simulink model "roboticSending"  (R2025b)
settings: Solver=FixedStepAuto  StartTime=0.0  StopTime=inf  RelTol=1e-3
model workspace (MAT data in the model file):
  SL_ROS_VariableLengthArrays_MaxSizes.CommonInfo.ArrayTruncateAction = 'EmitWarning'
  SL_ROS_VariableLengthArrays_MaxSizes.MsgTypeMap = containers.Map
  SL_ROS_VariableLengthArrays_MaxSizes.MsgTypeMap.serialization.keys = {'control_msgs/JointJog', 'sensor_msgs/JointState'}
  SL_ROS_VariableLengthArrays_MaxSizes.MsgTypeMap.serialization.values{1}(1).PropertyName = 'displacements'
  SL_ROS_VariableLengthArrays_MaxSizes.MsgTypeMap.serialization.values{1}(1).DataType = 'double'
  SL_ROS_VariableLengthArrays_MaxSizes.MsgTypeMap.serialization.values{1}(1).MaxLength = 6
  SL_ROS_VariableLengthArrays_MaxSizes.MsgTypeMap.serialization.values{1}(2).PropertyName = 'joint_names'
  SL_ROS_VariableLengthArrays_MaxSizes.MsgTypeMap.serialization.values{1}(2).DataType = 'std_msgs/String'
  SL_ROS_VariableLengthArrays_MaxSizes.MsgTypeMap.serialization.values{1}(2).MaxLength = 6
  SL_ROS_VariableLengthArrays_MaxSizes.MsgTypeMap.serialization.values{1}(3).PropertyName = 'velocities'
  SL_ROS_VariableLengthArrays_MaxSizes.MsgTypeMap.serialization.values{1}(3).DataType = 'double'
  SL_ROS_VariableLengthArrays_MaxSizes.MsgTypeMap.serialization.values{1}(3).MaxLength = 6
  SL_ROS_VariableLengthArrays_MaxSizes.MsgTypeMap.serialization.values{2}(1).PropertyName = 'effort'
  SL_ROS_VariableLengthArrays_MaxSizes.MsgTypeMap.serialization.values{2}(1).DataType = 'double'
  SL_ROS_VariableLengthArrays_MaxSizes.MsgTypeMap.serialization.values{2}(1).MaxLength = 6
  SL_ROS_VariableLengthArrays_MaxSizes.MsgTypeMap.serialization.values{2}(2).PropertyName = 'name'
  SL_ROS_VariableLengthArrays_MaxSizes.MsgTypeMap.serialization.values{2}(2).DataType = 'std_msgs/String'
  SL_ROS_VariableLengthArrays_MaxSizes.MsgTypeMap.serialization.values{2}(2).MaxLength = 6
  SL_ROS_VariableLengthArrays_MaxSizes.MsgTypeMap.serialization.values{2}(3).PropertyName = 'position'
  SL_ROS_VariableLengthArrays_MaxSizes.MsgTypeMap.serialization.values{2}(3).DataType = 'double'
  SL_ROS_VariableLengthArrays_MaxSizes.MsgTypeMap.serialization.values{2}(3).MaxLength = 6
  SL_ROS_VariableLengthArrays_MaxSizes.MsgTypeMap.serialization.values{2}(4).PropertyName = 'velocity'
  SL_ROS_VariableLengthArrays_MaxSizes.MsgTypeMap.serialization.values{2}(4).DataType = 'double'
  SL_ROS_VariableLengthArrays_MaxSizes.MsgTypeMap.serialization.values{2}(4).MaxLength = 6
  SL_ROS_VariableLengthArrays_MaxSizes.MsgTypeMap.serialization.uniformity = 0
  SL_ROS_VariableLengthArrays_MaxSizes.MsgTypeMap.serialization.keyType = 'char'
  SL_ROS_VariableLengthArrays_MaxSizes.MsgTypeMap.serialization.valueType = 'any'
values from neighbouring files (symbols this model uses):
  Error_threshold = 0.03    [RoboticCourseworkdata.sldd]
  Kd = 0.01    [RoboticCourseworkdata.sldd]
  Ki = 0.02    [RoboticCourseworkdata.sldd]
  Kp = 5.0    [RoboticCourseworkdata.sldd]
  Sample_time = 0.02    [RoboticCourseworkdata.sldd]
undefined symbols (not defined in the file or in its folder): DiscIntNeverNeededParam, Levenberg, Marquardt, velocities, velocities_SL_Info
libraries: ros2lib x3, robotmaniplib x2, robotcorelib x1, simulink_extras x1, simulink x1, SignalEditorBlockLib x1
settings Model: DataDictionary=RoboticCourseworkdata.sldd  Creator=jack  LastModifiedBy=jack
settings OptimizationCC: DefaultParameterBehavior=Inlined  EnhancedBackFolding=on  PassReuseOutputArgsAs=Individual arguments  ZeroExternalMemoryAtStartup=off  ZeroInternalMemoryAtStartup=off  MaxStackSize=64  OptimizeBlockOrder=speed  DifferentSizesBufferReuse=on  OptimizationCustomize=off  EfficientTunableParamExpr=on
settings DebuggingCC: ParameterTunabilityLossMsg=error
settings HardwareCC: ProdBitPerLong=64.0  ProdHWDeviceType=Intel->x86-64 (Linux 64)
settings SFSimCC: MATLABDynamicMemAlloc=off
settings RTWCC: SystemTargetFile=ert.tlc  HardwareBoard=Robot Operating System 2 (ROS 2)  TLCOptions="-aInlineSetEventsForThisBaseRateFcn=TLC_FALSE -aSuppressMultiTaskScheduler=TLC_FALSE  -aRateBasedStepFcn=0"  GenCodeOnly=on  TemplateMakefile=ert_default_tmf  Toolchain=Colcon Tools  TargetLang=C++  Description=Embedded Coder
settings CodeAppCC: ForceParamTrailComments=on  IgnoreCustomStorageClasses=off  OperatorAnnotations=on  SimulinkDataObjDesc=on  SFDataObjDesc=on  InsertBlockDesc=on
settings ERTTargetCC: ExtModeTransport=2.0  ExtModeStaticAlloc=on  ExtModeMexFile=ext_xcp  ExtModeIntrfLevel=Level2 - Open  RootIOFormat=Structure reference  CodeInterfacePackaging=C++ class

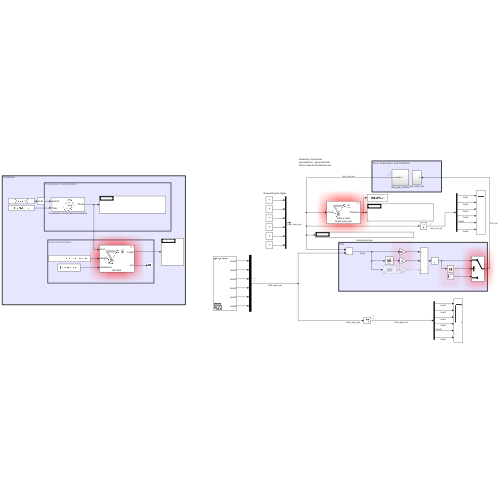
[thumbnail: Simulink's stored preview of the top-level diagram]
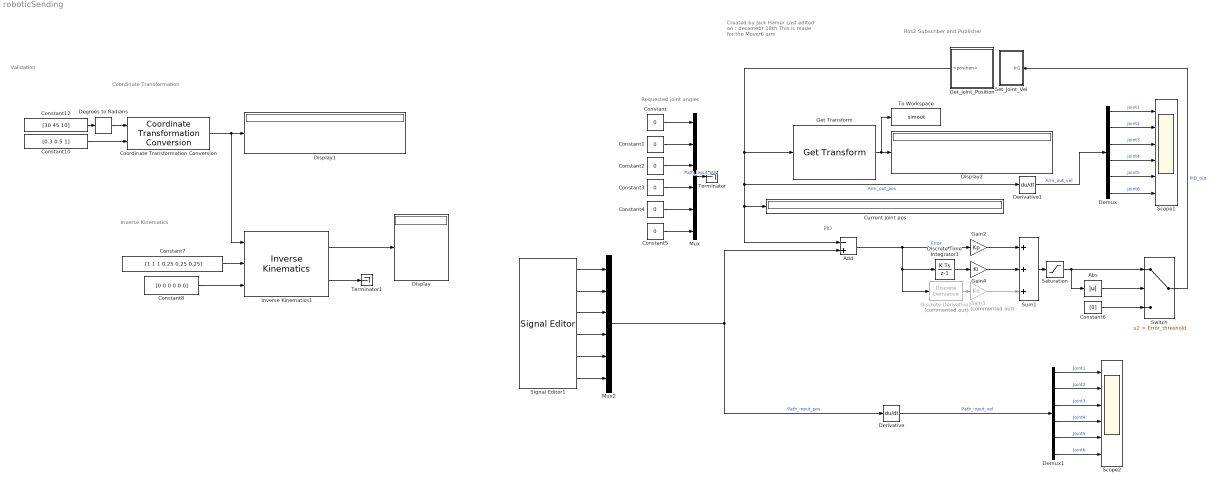
== system roboticSending ==
  note: Validation
  note: Created by Jack Hamer
      | Last edited on : decemebr 18th
      | This is made for the Mover6 arm
  note: Coordinate Transformation
  note: Inverse Kinematics
  note: PID
  note: Ros2 Subscriber and Publisher
  note: Requested joint angles
  Abs : Abs  SaturateOnIntegerOverflow=off
  Add : Sum  Inputs=-+
  Constant{,1..5} (6 alike) : Constant  Value=0
  Constant10 : Constant  Value=[0.3 0.5 1]
  Constant12 : Constant  Value=[30 45 10]
  Constant6 : Constant  Value=[0]  SampleTime=Sample_time
  Constant7 : Constant  Value=[1 1 1 0.25 0.25 0.25]
  Constant8 : Constant  Value=[0 0 0 0 0 0]
  Coordinate Transformation Conversion : robotcorelib/Coordinate Transformation Conversion  InputRepresentation=Euler Angles  InputEulerSequence=ZYX  ShowTrVecInputPort=on  OutputRepresentation=Homogeneous Transformation  OutputEulerSequence=ZYX  ShowTrVecOutputPort=on  SimulateUsing=Interpreted execution
  Current joint pos : Display
  Degrees to Radians : simulink_extras/Transformations/Degrees to Radians
  Demux : Demux  Outputs=6
  Demux1 : Demux  Outputs=6
  Derivative : Derivative
  Derivative1 : Derivative
  Discrete Derivative1 : simulink/Discrete/Discrete Derivative  Commented=on  gainval=1.0  ICPrevScaledInput=0.0  OutMin=[]  OutMax=[]  OutDataType=fixdt(1, 16)  OutScaling=2^-10  DoSatur=off
  Discrete-Time Integrator1 : DiscreteIntegrator  SampleTime=-1  ICPrevOutput=DiscIntNeverNeededParam  ICPrevScaledInput=DiscIntNeverNeededParam
  Display : Display
  Display1 : Display
  Display2 : Display
  Gain2 : Gain  Gain=Kp
  Gain3 : Gain  Commented=on  Gain=Kd
  Gain4 : Gain  Gain=Ki
  Get Transform : robotmaniplib/Get Transform  RigidBodyTree=Mover6import  SourceBody=link6  TargetBody=base_link  SimulateUsing=Interpreted execution
  Get_joint_Position : Subsystem
  Inverse Kinematics1 : robotmaniplib/Inverse Kinematics  RigidBodyTree=Mover6import  EndEffector=link6  ShowInfo=on  SolverName=Levenberg-Marquardt  EnforceJointLimits=on  MaxIterations=1500  MaxTime=10  GradientTolerance=1e-3  SolutionTolerance=1e-2  StepTolerance=1e-7  ConstraintTolerance=1e-6  ErrorChangeTolerance=1e-3  UseErrorDamping=on  DampingBias=0.0025  SimulateUsing=Interpreted execution
  Mux : Mux  Inputs=6
  Mux2 : Mux  Inputs=6
  Saturation : Saturate  UpperLimit=2  LowerLimit=-2
  Scope1 : Scope  NumInputPorts=6
      settings: ActiveDisplayYMinimum=-3.329826235975621  ActiveDisplayYMaximum=3.372443564924636
  Scope2 : Scope  NumInputPorts=6
      settings: ActiveDisplayYMinimum=-1.9531250848653292  ActiveDisplayYMaximum=2.2527181340884104
  Set_Joint_Vel : Subsystem
  Signal Editor1 : SignalEditorBlockLib/Signal Editor  FileName=TrapzodialControlsig.mat  ActiveScenario=path_senario  ActiveSignal=Joint1  IsBus=off  OutputBusObjectStr=Bus: BusObject  SampleTime=0  ZeroCross=off  OutputAfterFinalValue=Holding final value  Unit=inherit  PreserveSignalName=on  ApplySigPropsToAllScenarios=on  ApplySigPropsToAllSignals=on  SignalPropertySource=Dialog parameters
  Sum1 : Sum  Inputs=+++
  Switch : Switch  Criteria=u2 > Threshold  Threshold=Error_threshold  SaturateOnIntegerOverflow=off  InputSameDT=off
  Terminator : Terminator
  Terminator1 : Terminator
  To Workspace : ToWorkspace  VariableName=simout  SaveFormat=Timeseries  SampleTime=-1
  wires:
  Saturation/1 -> Switch/1, Abs/1
  Sum1/1 -> Saturation/1
  Gain2/1 -> Sum1/1
  Add/1 -> Discrete Derivative1/1, Discrete-Time Integrator1/1, Gain2/1  "Error"
  Discrete-Time Integrator1/1 -> Gain4/1
  Gain4/1 -> Sum1/2
  Gain3/1 -> Sum1/3
  Discrete Derivative1/1 -> Gain3/1
  Constant/1 -> Mux/1
  Constant1/1 -> Mux/2
  Constant2/1 -> Mux/3
  Constant5/1 -> Mux/6
  Constant4/1 -> Mux/5
  Constant3/1 -> Mux/4
  Abs/1 -> Switch/2
  Constant6/1 -> Switch/3
  Demux/1 -> Scope1/1  "Joint1"
  Demux/2 -> Scope1/2  "Joint2"
  Demux/3 -> Scope1/3  "Joint3"
  Demux/4 -> Scope1/4  "Joint4"
  Demux/6 -> Scope1/6  "Joint6"
  Demux/5 -> Scope1/5  "Joint5"
  Inverse Kinematics1/2 -> Terminator1/1
  Coordinate Transformation Conversion/1 -> Inverse Kinematics1/1, Display1/1
  Constant7/1 -> Inverse Kinematics1/2
  Constant8/1 -> Inverse Kinematics1/3
  Inverse Kinematics1/1 -> Display/1
  Get Transform/1 -> To Workspace/1, Display2/1
  Switch/1 -> Set_Joint_Vel/1(In1)  "PID_out"
  Degrees to Radians/1 -> Coordinate Transformation Conversion/1
  Signal Editor1/1 -> Mux2/1
  Signal Editor1/2 -> Mux2/2
  Signal Editor1/3 -> Mux2/3
  Signal Editor1/4 -> Mux2/4
  Signal Editor1/5 -> Mux2/5
  Signal Editor1/6 -> Mux2/6
  Constant12/1 -> Degrees to Radians/1
  Constant10/1 -> Coordinate Transformation Conversion/2
  Demux1/5 -> Scope2/5  "Joint5"
  Demux1/6 -> Scope2/6  "Joint6"
  Demux1/4 -> Scope2/4  "Joint4"
  Demux1/3 -> Scope2/3  "Joint3"
  Demux1/2 -> Scope2/2  "Joint2"
  Demux1/1 -> Scope2/1  "Joint1"
  Derivative/1 -> Demux1/1  "Path_input_vel"
  Get_joint_Position/1(<position>) -> Get Transform/1, Derivative1/1, Add/1, Current joint pos/1  "Arm_out_pos"
  Derivative1/1 -> Demux/1  "Arm_out_vel"
  Mux2/1 -> Add/2, Derivative/1  "Path_input_pos"
  Mux/1 -> Terminator/1  "Path_input_pos"

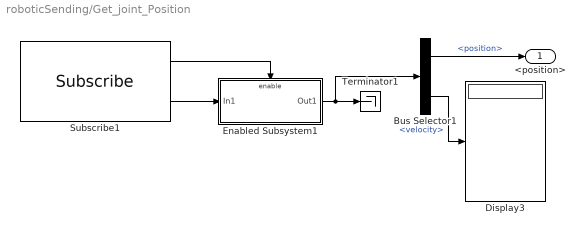
== system roboticSending/Get_joint_Position ==
  Bus Selector1 : BusSelector  OutputSignals=position,velocity
  Display3 : Display
  Enabled Subsystem1 : Subsystem  TreatAsAtomicUnit=on
  Subscribe1 : ros2lib/Subscribe  topicSource=Select from ROS network  topic=/joint_states  messageType=sensor_msgs/JointState  sampleTime=Sample_time  QOSHistory=Keep last  QOSDepth=10  QOSReliability=Reliable  QOSDurability=Volatile  QOSDeadline=Inf  QOSLifespan=Inf  QOSLiveliness=Automatic  QOSLeaseDuration=Inf  QOSAvoidROSNamespaceConventions=off
  Terminator1 : Terminator
  <position> : Outport
  wires:
  Subscribe1/1 -> Enabled Subsystem1/Enable
  Subscribe1/2 -> Enabled Subsystem1/1(In1)
  Bus Selector1/2 -> Display3/1  "<velocity>"
  Enabled Subsystem1/1(Out1) -> Bus Selector1/1, Terminator1/1
  Bus Selector1/1 -> <position>/1  "<position>"

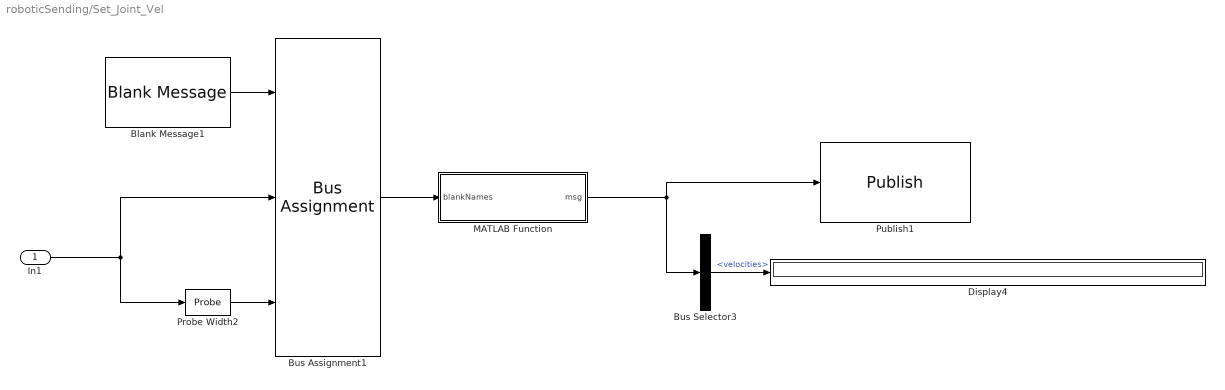
== system roboticSending/Set_Joint_Vel ==
  In1 : Inport
  Blank Message1 : ros2lib/Blank Message  messageClass=Message  entityType=control_msgs/JointJog  messageType=control_msgs/JointJog  SampleTime=Sample_time
  Bus Assignment1 : BusAssignment  AssignedSignals=velocities,velocities_SL_Info.CurrentLength
  Bus Selector3 : BusSelector  OutputSignals=velocities
  Display4 : Display
  MATLAB Function : MATLAB Function  TreatAsAtomicUnit=on
  Probe Width2 : Probe  ProbeSampleTime=off  ProbeComplexSignal=off  ProbeWidthDataType=uint32
  Publish1 : ros2lib/Publish  topicSource=Select from ROS network  topic=/JointJog  messageType=control_msgs/JointJog  QOSHistory=Keep last  QOSDepth=10  QOSReliability=Reliable  QOSDurability=Volatile  QOSDeadline=Inf  QOSLifespan=Inf  QOSLiveliness=Automatic  QOSLeaseDuration=Inf  QOSAvoidROSNamespaceConventions=off
  wires:
  Bus Assignment1/1 -> MATLAB Function/1(blankNames)
  Probe Width2/1 -> Bus Assignment1/3
  Bus Selector3/1 -> Display4/1  "<velocities>"
  In1/1 -> Bus Assignment1/2, Probe Width2/1
  Blank Message1/1 -> Bus Assignment1/1
  MATLAB Function/1(msg) -> Publish1/1, Bus Selector3/1

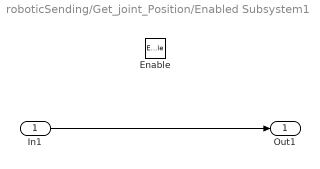
== system roboticSending/Get_joint_Position/Enabled Subsystem1 ==
  In1 : Inport
  Enable : EnablePort
  Out1 : Outport
  wires:
  In1/1 -> Out1/1

== matlab function roboticSending/Set_Joint_Vel/MATLAB Function ==
  data: blankNames input; msg output Bus: SL_Bus_control_msgs_JointJog
function msg = addsnamestobus(blankNames)
%Very heavily edited from The matworks string ros2 assigment script
%https://uk.mathworks.com/help/ros/ug/work-with-ros2-messages-in-simulink.html
% specifically the working with string assignment example

strArraytoinput={'joint1','joint2','joint3','joint4','joint5','joint6'};

msg=blankNames;

lenofarray=length(strArraytoinput);

msg.joint_names_SL_Info.CurrentLength=uint32(lenofarray);


for idx=1:lenofarray
    str = strArraytoinput{idx};
    strLength = length(str);
    msg.joint_names(idx).data(1:strLength) = uint8(str);
    msg.joint_names(idx).data_SL_Info.CurrentLength = uint32(strLength);
end
